simulink model "FOC_test1"  (R2022b)
settings: Solver=FixedStepAuto  StartTime=0.0  StopTime=2  FixedStep=1e-6  RelTol=1e-3
libraries: simulink x2, spsDCVoltageSourceLib x1, spsPermanentMagnetSynchronousMachineLib x1, spsTwoLevelConverterLib x1, spspowerguiLib x1
settings Model: Creator=User  LastModifiedBy=Mengyang

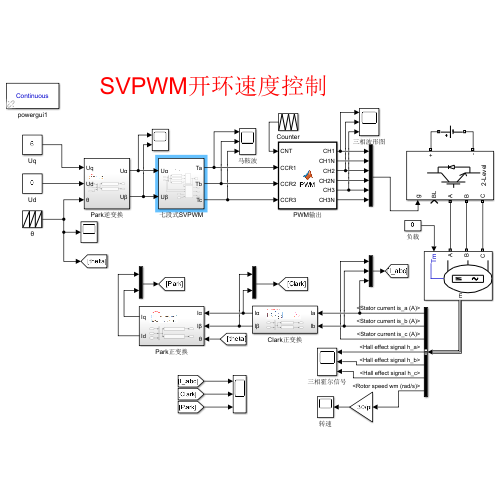
[thumbnail: Simulink's stored preview of the top-level diagram]
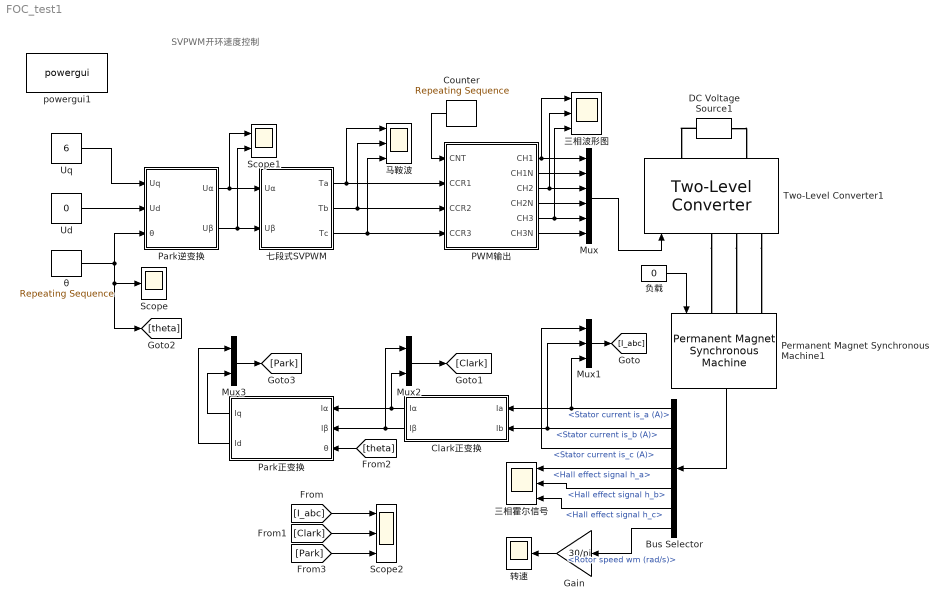
== system FOC_test1 ==
  note: SVPWM开环速度控制
  Bus Selector : BusSelector  OutputSignals=Stator current is_a (A),Stator current is_b (A),Stator current is_c (A),Hall effect signal h_a,Hall effect signal h_b,Hall effect signal h_c,Rotor speed wm (rad/s)
  Clark正变换 : Subsystem
  Counter : simulink/Sources/Repeating Sequence  rep_seq_t=[0 0.00005 0.0001]  rep_seq_y=[0 100 1]
  DC Voltage Source1 : spsDCVoltageSourceLib/DC Voltage Source  Amplitude=12  Measurements=None
  Gain : Gain  Gain=30/pi
  Mux : Mux  Inputs=6
  Mux1 : Mux  Inputs=3
  Mux2 : Mux  Inputs=2
  Mux3 : Mux  Inputs=2
  PWM输出 : MATLAB Function  TreatAsAtomicUnit=on
  Park正变换 : Subsystem
  Park逆变换 : Subsystem
  Permanent Magnet Synchronous Machine1 : spsPermanentMagnetSynchronousMachineLib/Permanent Magnet Synchronous Machine  NbPhases=3  FluxDistribution=Sinusoidal  RotorType=Round  MechanicalLoad=Torque Tm  PresetModel=No  ShowDetailedParameters=on  MeasurementBus=off  Resistance=0.0485  Inductance=8.5e-3  dqInductances=[8.5e-3,8.5e-3]  La=0.000395  MachineConstant=Flux linkage established by magnets (V.s)  Flux=0.1194  VoltageCst=86.6271  TorqueCst=0.7164  Flat=120  Mechanical=[0.0027 0.0004924 4 0]  PolePairs=4  InitialConditions=[0,0, 0,0]  InitialConditions5ph=[0 0 0 0 0 0]  RefAngle=Aligned with phase A axis (original Park)  IterativeDiscreteModel=Trapezoidal non iterative  TsBlock=-1  TsPowergui=0
  Scope : Scope
  Scope1 : Scope  NumInputPorts=2
  Scope2 : Scope  NumInputPorts=3
  Two-Level Converter1 : spsTwoLevelConverterLib/Two-Level Converter  ModelType=Switching devices  Ron=1e-3  Rs=1e6  Cs=inf  Vforward=[0,0]  Ron_Diode=1e-3  Rs_Diode=1e6  Cs_Diode=inf  Vf_Diode=1e-3  Rs_CurrentSource=inf  Ron_ACsource=1e-3
  Ud : Constant  Value=0
  Uq : Constant  Value=6
  powergui1 : spspowerguiLib/powergui  Priority=1  SimulationMode=Continuous  SampleTime=0.000001  frequency=60  Iterations=50  frequencyindice=0  Pbase=100e6  ErrMax=1e-4  UnitsV=kV  UnitsW=MW  buscounter=0  FunctionMessages=off  echomessages=off  EnableUseOfTLC=off  CurrentSourceSwitches=off  DisableSnubberDevices=off  DisableRonSwitches=off  DisableVfSwitches=off  DisplayEquations=off  AutomaticDiscreteSolvers=off  SolverType=Tustin/Backward Euler (TBE)  Interpol=off  ExternalGateDelay=off  methode=off  Ts=100  x0status=blocks  SPID=on  SwTol=0  HookPort=off  NonlinearTolerance=1e-4  nMaxIteration=100  ContinueOnMaxIteration=off  RestoreLinks=warning  ResistiveCurrentMeasurement=off  Frange=[0:2:500]  Ylog=off  Xlog=on  ShowGrid=off  save=off  variable=ZData  structure=0  ZoomFFT=off  StartTime=0.0  cycles=1  DisplayStyle=1  fundamental=60  FreqAxis=off  MaxFrequency=1000  frequencyindicesteady=1  RmsSteady=1  display=off
  θ : simulink/Sources/Repeating Sequence  rep_seq_t=[0 1]  rep_seq_y=[0 2*pi]
  七段式SVPWM : Subsystem
  三相波形图 : Scope  NumInputPorts=3
  三相霍尔信号 : Scope  NumInputPorts=3
  负载 : Constant  Value=0
  转速 : Scope
  马鞍波 : Scope  NumInputPorts=3
  wires:
  Ud/1 -> Park逆变换/2(Ud)
  Uq/1 -> Park逆变换/1(Uq)
  Park逆变换/1(Uα) -> 七段式SVPWM/1(Uα), Scope1/1
  Park逆变换/2(Uβ) -> 七段式SVPWM/2(Uβ), Scope1/2
  七段式SVPWM/1(Ta) -> PWM输出/2(CCR1), 马鞍波/1
  七段式SVPWM/2(Tb) -> 马鞍波/2, PWM输出/3(CCR2)
  七段式SVPWM/3(Tc) -> PWM输出/4(CCR3), 马鞍波/3
  Counter/1 -> PWM输出/1(CNT)
  PWM输出/1(CH1) -> 三相波形图/1, Mux/1
  PWM输出/2(CH1N) -> Mux/2
  PWM输出/3(CH2) -> 三相波形图/2, Mux/3
  PWM输出/4(CH2N) -> Mux/4
  PWM输出/5(CH3) -> 三相波形图/3, Mux/5
  PWM输出/6(CH3N) -> Mux/6
  Mux/1 -> Two-Level Converter1/1
  负载/1 -> Permanent Magnet Synchronous Machine1/1
  Permanent Magnet Synchronous Machine1/1 -> Bus Selector/1
  Mux1/1 -> [I_abc]
  Bus Selector/1 -> Clark正变换/1(Ia), Mux1/3  "<Stator current is_a (A)>"
  Bus Selector/2 -> Clark正变换/2(Ib), Mux1/2  "<Stator current is_b (A)>"
  Bus Selector/3 -> Mux1/1  "<Stator current is_c (A)>"
  [I_abc] -> Scope2/1
  Clark正变换/2(Iβ) -> Park正变换/2(Iβ), Mux2/1
  Mux2/1 -> [Clark]
  [Clark] -> Scope2/2
  Clark正变换/1(Iα) -> Park正变换/1(Iα), Mux2/2
  [theta] -> Park正变换/3(θ)
  Park正变换/1(Iq) -> Mux3/2
  Park正变换/2(Id) -> Mux3/1
  Mux3/1 -> [Park]
  [Park] -> Scope2/3
  Bus Selector/4 -> 三相霍尔信号/1  "<Hall effect signal h_a>"
  Bus Selector/5 -> 三相霍尔信号/2  "<Hall effect signal h_b>"
  Bus Selector/6 -> 三相霍尔信号/3  "<Hall effect signal h_c>"
  Gain/1 -> 转速/1
  Bus Selector/7 -> Gain/1  "<Rotor speed wm (rad/s)>"
  θ/1 -> Park逆变换/3(θ), Scope/1, [theta]
  connections:
  DC Voltage Source1/RConn1 -- Two-Level Converter1/RConn1
  DC Voltage Source1/LConn1 -- Two-Level Converter1/RConn2
  Two-Level Converter1/LConn1 -- Permanent Magnet Synchronous Machine1/LConn1
  Two-Level Converter1/LConn2 -- Permanent Magnet Synchronous Machine1/LConn2
  Two-Level Converter1/LConn3 -- Permanent Magnet Synchronous Machine1/LConn3

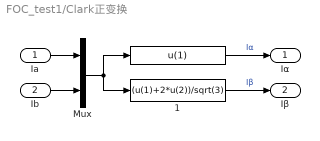
== system FOC_test1/Clark正变换 ==
  Ia : Inport
  Ib : Inport  Port=2
  " " : Fcn  Expr=u(1)
  " 1" : Fcn  Expr=(u(1)+2*u(2))/sqrt(3)
  Mux : Mux  Inputs=2
  Iα : Outport
  Iβ : Outport  Port=2
  wires:
  Ia/1 -> Mux/1
  Ib/1 -> Mux/2
  " "/1 -> Iα/1  "Iα"
  " 1"/1 -> Iβ/1  "Iβ"
  Mux/1 -> " 1"/1, " "/1

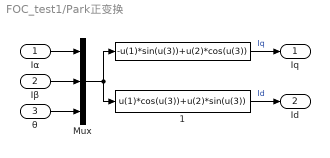
== system FOC_test1/Park正变换 ==
  Iα : Inport
  Iβ : Inport  Port=2
  θ : Inport  Port=3
  " " : Fcn  Expr=-u(1)*sin(u(3))+u(2)*cos(u(3))
  " 1" : Fcn  Expr=u(1)*cos(u(3))+u(2)*sin(u(3))
  Mux : Mux  Inputs=3
  Iq : Outport
  Id : Outport  Port=2
  wires:
  Iα/1 -> Mux/1
  Iβ/1 -> Mux/2
  " "/1 -> Iq/1  "Iq"
  " 1"/1 -> Id/1  "Id"
  Mux/1 -> " "/1, " 1"/1
  θ/1 -> Mux/3

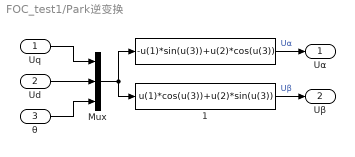
== system FOC_test1/Park逆变换 ==
  Uq : Inport
  Ud : Inport  Port=2
  θ : Inport  Port=3
  " " : Fcn  Expr=-u(1)*sin(u(3))+u(2)*cos(u(3))
  " 1" : Fcn  Expr=u(1)*cos(u(3))+u(2)*sin(u(3))
  Mux : Mux  Inputs=3
  Uα : Outport
  Uβ : Outport  Port=2
  wires:
  Ud/1 -> Mux/2
  Uq/1 -> Mux/1
  θ/1 -> Mux/3
  " 1"/1 -> Uβ/1  "Uβ"
  " "/1 -> Uα/1  "Uα"
  Mux/1 -> " 1"/1, " "/1

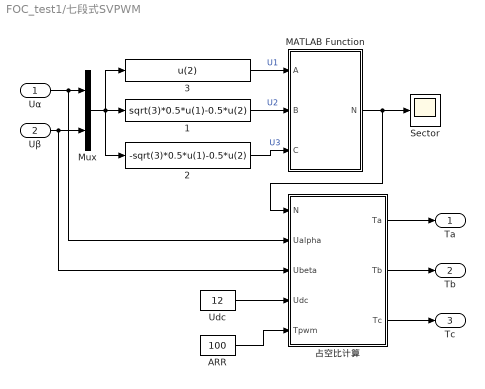
== system FOC_test1/七段式SVPWM ==
  Uα : Inport
  Uβ : Inport  Port=2
  " 1" : Fcn  Expr=sqrt(3)*0.5*u(1)-0.5*u(2)
  " 2" : Fcn  Expr=-sqrt(3)*0.5*u(1)-0.5*u(2)
  " 3" : Fcn  Expr=u(2)
  ARR : Constant  Value=100
  MATLAB Function : MATLAB Function  TreatAsAtomicUnit=on
  Mux : Mux  Inputs=2
  Sector : Scope
  Udc : Constant  Value=12
  占空比计算 : MATLAB Function  TreatAsAtomicUnit=on
  Ta : Outport
  Tb : Outport  Port=2
  Tc : Outport  Port=3
  wires:
  Uα/1 -> 占空比计算/2(Ualpha), Mux/1
  Uβ/1 -> 占空比计算/3(Ubeta), Mux/2
  Mux/1 -> " 2"/1, " 3"/1, " 1"/1
  " 3"/1 -> MATLAB Function/1(A)  "U1"
  " 1"/1 -> MATLAB Function/2(B)  "U2"
  " 2"/1 -> MATLAB Function/3(C)  "U3"
  MATLAB Function/1(N) -> 占空比计算/1(N), Sector/1
  Udc/1 -> 占空比计算/4(Udc)
  ARR/1 -> 占空比计算/5(Tpwm)
  占空比计算/1(Ta) -> Ta/1
  占空比计算/2(Tb) -> Tb/1
  占空比计算/3(Tc) -> Tc/1

== matlab function FOC_test1/七段式SVPWM/占空比计算 ==
  data: N input; Ta output; Ualpha input; Ubeta input; Udc input; Tpwm input; Tb output; Tc output
function [Ta,Tb,Tc] = DutyCalculate(N,Ualpha,Ubeta,Udc,Tpwm)

Ta=double(0);
Tb=double(0);
Tc=double(0);

K = sqrt(3)*Tpwm/Udc;
U1 = Ubeta*K;
U2 = (sqrt(3)*Ualpha/2 - 0.5 * Ubeta)*K;
U3 = (-sqrt(3)*Ualpha/2 - 0.5 * Ubeta)*K;

%% 扇区1
if(N==3)  
   T4 = U2;
   T6 = U1;
   SUM = T4+T6;
   if(SUM>Tpwm)
       K_SVPWM = Tpwm/SUM;
       T4= K_SVPWM*T4;
       T6= K_SVPWM*T6;
   end
   T7=(Tpwm-T4-T6)/2;
   Ta = T4+T6+T7;
   Tb = T6+T7;
   Tc = T7;
end
%% 扇区2
if(N==1)  
   T2 = -U2;
   T6 = -U3;
   SUM = T2+T6;
   if(SUM>Tpwm)
       K_SVPWM = Tpwm/SUM;
       T2= K_SVPWM*T2;
       T6= K_SVPWM*T6;
   end
   T7=(Tpwm-T2-T6)/2;
   Ta = T6+T7;
   Tb = T2+T6+T7;
   Tc = T7;
end
%% 扇区3
if(N==5)  
   T2 = U1;
   T3 = U3;
   SUM = T2+T3;
   if(SUM>Tpwm)
       K_SVPWM = Tpwm/SUM;
       T2= K_SVPWM*T2;
       T3= K_SVPWM*T3;
   end
   T7=(Tpwm-T2-T3)/2;
   Ta = T7;
   Tb = T2+T3+T7;
   Tc = T3+T7;
end
%% 扇区4
if(N==4)  
   T1 = -U1;
   T3 = -U2;
   SUM = T1+T3;
   if(SUM>Tpwm)
       K_SVPWM = Tpwm/SUM;
       T1= K_SVPWM*T1;
       T3= K_SVPWM*T3;
   end
   T7=(Tpwm-T1-T3)/2;
   Ta = T7;
   Tb = T3+T7;
   Tc = T1+T3+T7;
end
%% 扇区5
if(N==6)  
   T1 = U3;
   T5 = U2;
   SUM = T1+T5;
   if(SUM>Tpwm)
       K_SVPWM = Tpwm/SUM;
       T1= K_SVPWM*T1;
       T5= K_SVPWM*T5;
   end
   T7=(Tpwm-T1-T5)/2;
   Ta = T5+T7;
   Tb = T7;
   Tc = T1+T5+T7;
end
%% 扇区6
if(N==2)  
   T4 = -U3;
   T5 = -U1;
   SUM = T4+T5;
   if(SUM>Tpwm)
       K_SVPWM = Tpwm/SUM;
       T4= K_SVPWM*T4;
       T5= K_SVPWM*T5;
   end
   T7=(Tpwm-T4-T5)/2;
   Ta = T4+T5+T7;
   Tb = T7;
   Tc = T5+T7;
end

== matlab function FOC_test1/七段式SVPWM/MATLAB Function ==
  data: A input; N output; B input; C input
function N = SectorJudge(A,B,C)
N=0;

% N = A + 2B + 4C
if(A>0)
    N=N+1;
end

if(B>0)
    N=N+2;
end

if(C>0)
    N=N+4;
end

== matlab function FOC_test1/PWM输出 ==
  data: CNT input; CH1 output; CCR1 input; CCR2 input; CCR3 input; CH1N output; CH2 output; CH2N output; CH3 output; CH3N output
function [CH1,CH1N,CH2,CH2N,CH3,CH3N] = PWM(CNT,CCR1,CCR2,CCR3)

if(CNT <= CCR1)
    CH1=0;
    CH1N=1;
else
    CH1=1;
    CH1N=0;
end

if(CNT <= CCR2)
    CH2=0;
    CH2N=1;
else
    CH2=1;
    CH2N=0;
end

if(CNT <= CCR3)
    CH3=0;
    CH3N=1;
else
    CH3=1;
    CH3N=0;
end
